simulink model "Adaptive_Control_Kd"  (R2021b)
settings: Solver=VariableStepAuto  StartTime=0.0  StopTime=50  RelTol=1e-3
undefined symbols (not defined in the file or in its folder): Kd, Kpi, Lambda, q_dq_init
(part 1 of 4)
settings Model: Creator=Yafei Ou  LastModifiedBy=Yafei Ou

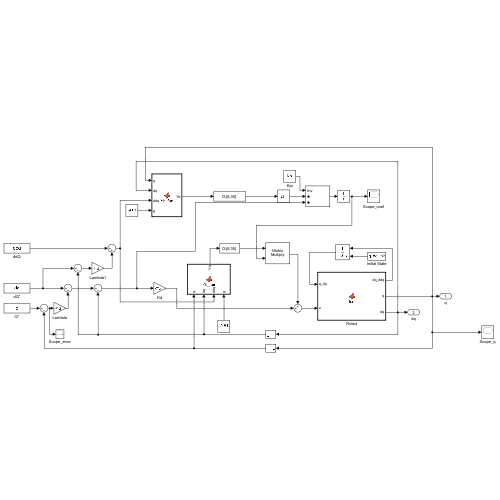
[thumbnail: Simulink's stored preview of the top-level diagram]
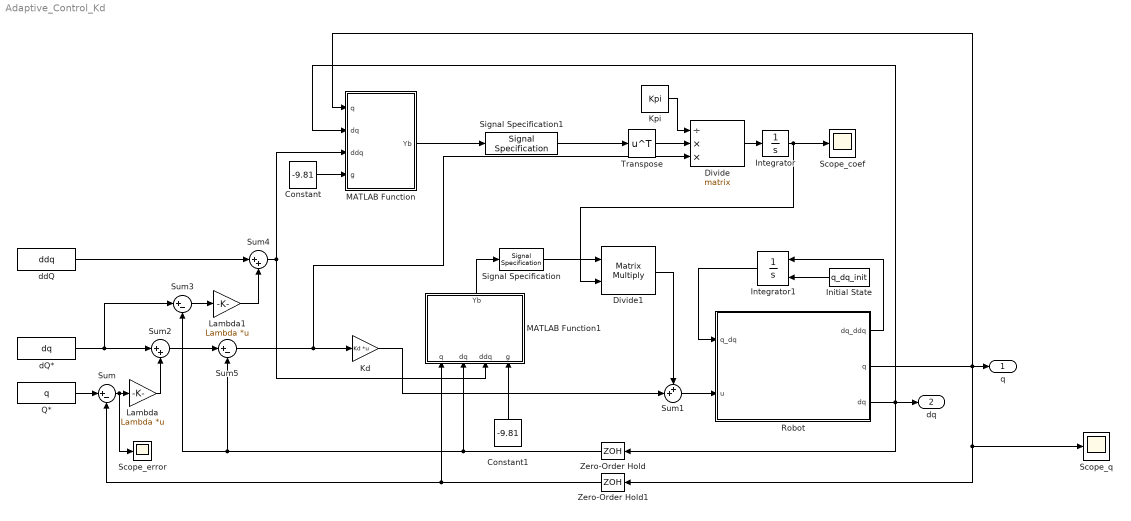
== system Adaptive_Control_Kd ==
  Constant : Constant  Value=-9.81
  Constant1 : Constant  Value=-9.81
  Divide : Product  Inputs=/**  Multiplication=Matrix(*)
  Divide1 : Product  Multiplication=Matrix(*)
  Initial State : Constant  Value=q_dq_init
  Integrator : Integrator
  Integrator1 : Integrator  InitialConditionSource=external
  Kd : Gain  Gain=Kd  Multiplication=Matrix(K*u)
  Kpi : Constant  Value=Kpi
  Lambda : Gain  Gain=Lambda  Multiplication=Matrix(K*u)
  Lambda1 : Gain  Gain=Lambda  Multiplication=Matrix(K*u)
  MATLAB Function : MATLAB Function  TreatAsAtomicUnit=on
  MATLAB Function1 : MATLAB Function  TreatAsAtomicUnit=on
  Q* : FromWorkspace  VariableName=q
  Robot : MATLAB Function  TreatAsAtomicUnit=on
  Scope_coef : Scope
  Scope_error : Scope
  Scope_q : Scope
  Signal Specification : SignalSpecification  Dimensions=[6,35]
  Signal Specification1 : SignalSpecification  Dimensions=[6,35]
  Sum : Sum  Inputs=|+-
  Sum1 : Sum  Inputs=++|
  Sum2 : Sum  Inputs=|++
  Sum3 : Sum  Inputs=|+-
  Sum4 : Sum  Inputs=|++
  Sum5 : Sum  Inputs=|+-
  Transpose : Math  Operator=transpose  SaturateOnIntegerOverflow=on
  Zero-Order Hold : ZeroOrderHold  SampleTime=0.001
  Zero-Order Hold1 : ZeroOrderHold  SampleTime=0.001
  dQ* : FromWorkspace  VariableName=dq
  ddQ : FromWorkspace  VariableName=ddq
  q : Outport
  dq : Outport  Port=2
  wires:
  Sum1/1 -> Robot/2(u)
  Q*/1 -> Sum/1
  Robot/2(q) -> Scope_q/1, Zero-Order Hold1/1, MATLAB Function/1(q), q/1
  Robot/3(dq) -> MATLAB Function/2(dq), Zero-Order Hold/1, dq/1
  Robot/1(dq_ddq) -> Integrator1/1
  Integrator1/1 -> Robot/1(q_dq)
  Initial State/1 -> Integrator1/2
  Constant/1 -> MATLAB Function/4(g)
  Sum/1 -> Scope_error/1, Lambda/1
  Lambda/1 -> Sum2/2
  dQ*/1 -> Sum3/1, Sum2/1
  Sum3/1 -> Lambda1/1
  ddQ/1 -> Sum4/1
  Lambda1/1 -> Sum4/2
  MATLAB Function/1(Yb) -> Signal Specification1/1
  Transpose/1 -> Divide/2
  Sum4/1 -> MATLAB Function/3(ddq), MATLAB Function1/3(ddq)
  Kpi/1 -> Divide/1
  Divide/1 -> Integrator/1
  Constant1/1 -> MATLAB Function1/4(g)
  Sum2/1 -> Sum5/1
  Kd/1 -> Sum1/2
  Signal Specification/1 -> Divide1/1
  Sum5/1 -> Kd/1, Divide/3
  Divide1/1 -> Sum1/1
  Integrator/1 -> Divide1/2, Scope_coef/1
  MATLAB Function1/1(Yb) -> Signal Specification/1
  Signal Specification1/1 -> Transpose/1
  Zero-Order Hold/1 -> Sum5/2, Sum3/2, MATLAB Function1/2(dq)
  Zero-Order Hold1/1 -> MATLAB Function1/1(q), Sum/2
